simulink model "mmt_klo_continious_1"  (Simulink 7.6)
settings: Solver=ode45  StartTime=0.0  StopTime=10.0  FixedStep=0.1  MaxStep=0.1  RelTol=1e-3
undefined symbols (not defined in the file or in its folder): A, B, p
settings Model: Creator=Stuffy  LastModifiedBy=Stuffy

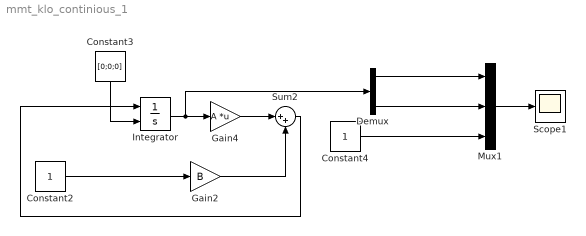
== system mmt_klo_continious_1 ==
  Constant2 : Constant
  Constant3 : Constant  Value=[0;0;0]  VectorParams1D=off
  Constant4 : Constant
  Demux : Demux  Outputs=3
  Gain2 : Gain  Gain=B
  Gain4 : Gain  Gain=A  Multiplication=Matrix(K*u)
  Integrator : Integrator  InitialConditionSource=external  InitialCondition=p
  Mux1 : Mux  Inputs=3
  Scope1 : Scope
  Sum2 : Sum  Inputs=|++
  wires:
  Gain2/1 -> Sum2/2
  Constant2/1 -> Gain2/1
  Constant3/1 -> Integrator/2
  Integrator/1 -> Gain4/1, Demux/1
  Gain4/1 -> Sum2/1
  Sum2/1 -> Integrator/1
  Mux1/1 -> Scope1/1
  Demux/1 -> Mux1/1
  Demux/3 -> Mux1/2
  Constant4/1 -> Mux1/3
